simulink model "TestWindRacingDynamicModelRealForce"  (R2022b)
settings: Solver=FixedStepAuto  StartTime=0.0  StopTime=137  FixedStep=simulator.TimeStep  RelTol=1e-3
undefined symbols (not defined in the file): simulator
settings Model: Creator=At  LastModifiedBy=ateay
settings SolverCC: ConcurrentTasks=on  AlgebraicLoopSolver=TrustRegion  InsertRTBMode=Never (minimum delay)
settings DataIOCC: ReturnWorkspaceOutputs=off
settings DebuggingCC: UnconnectedInputMsg=warning  UnconnectedOutputMsg=warning  UnconnectedLineMsg=warning  SFMachineParentedDataDiag=warning  ArithmeticOperatorsInVariantConditions=warning
settings ModelReferenceCC: EnableRefExpFcnMdlSchedulingChecks=on
settings SFSimCC: SimUseLocalCustomCode=off  CustomCodeUndefinedFunction=UseInterfaceOnly
settings RTWCC: RTWUseLocalCustomCode=off
settings CodeAppCC: StateflowObjectComments=on

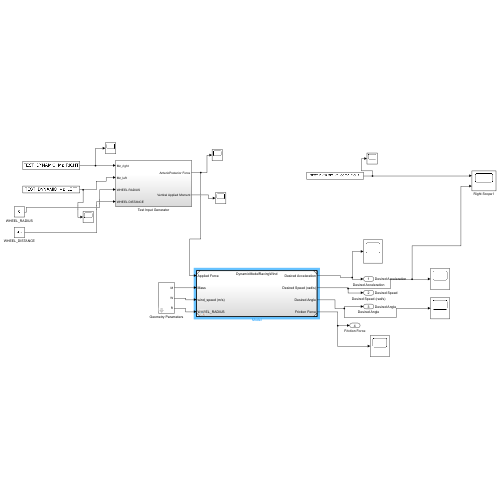
[thumbnail: Simulink's stored preview of the top-level diagram]
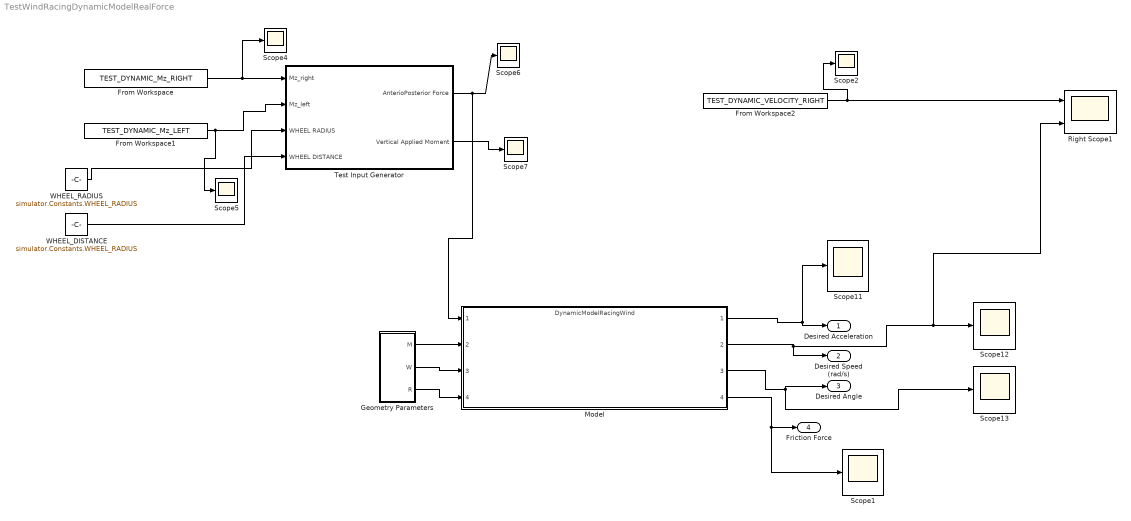
== system TestWindRacingDynamicModelRealForce ==
  From Workspace : FromWorkspace  VariableName=TEST_DYNAMIC_Mz_RIGHT
  From Workspace1 : FromWorkspace  VariableName=TEST_DYNAMIC_Mz_LEFT
  From Workspace2 : FromWorkspace  VariableName=TEST_DYNAMIC_VELOCITY_RIGHT
  Geometry Parameters : Subsystem  mask{M=simulator.Sim.Dynamics.Mass, W=simulator.Sim.Dynamics.wind_speed, rR=simulator.Constants.WHEEL_RADIUS}
      mask prompts: M "Mass"; W "Wind"; rR "Radius"
      mask TypeOptions M: Mass/Value
      mask TypeOptions rR: rR/Value
  Model : ModelReference  ModelNameDialog=DynamicModelRacingWind.slx  SimulationMode=Normal  ModelReferenceVersion=1.17
  Right Scope1 : Scope  NumInputPorts=2
  Scope{1..2,4..7,11..13} (9 alike) : Scope
  Test Input Generator : Subsystem
  WHEEL_DISTANCE : Constant  Value=simulator.Constants.WHEEL_RADIUS
  WHEEL_RADIUS : Constant  Value=simulator.Constants.WHEEL_RADIUS
  Desired Acceleration : Outport  SignalName=Desired Acceleration
  Desired Speed (rad/s) : Outport  Port=2  SignalName=Desired Speed
  Desired Angle : Outport  Port=3  SignalName=Desired Angle
  Friction Force : Outport  Port=4
  wires:
  WHEEL_RADIUS/1 -> Test Input Generator/3(WHEEL RADIUS)
  WHEEL_DISTANCE/1 -> Test Input Generator/4(WHEEL DISTANCE)
  Test Input Generator/1(AnterioPosterior Force) -> Scope6/1, Model/1
  Test Input Generator/2(Vertical Applied Moment) -> Scope7/1
  From Workspace/1 -> Scope4/1, Test Input Generator/1(Mz_right)
  From Workspace1/1 -> Scope5/1, Test Input Generator/2(Mz_left)
  From Workspace2/1 -> Scope2/1, Right Scope1/1
  Geometry Parameters/1(M) -> Model/2
  Geometry Parameters/2(W) -> Model/3
  Geometry Parameters/3(R) -> Model/4
  Model/3 -> Desired Angle/1, Scope13/1
  Model/2 -> Desired Speed (rad/s)/1, Right Scope1/2, Scope12/1
  Model/1 -> Desired Acceleration/1, Scope11/1
  Model/4 -> Scope1/1, Friction Force/1

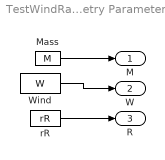
== system TestWindRacingDynamicModelRealForce/Geometry Parameters ==
  Mass : Constant  Value=M
  Wind : Constant  Value=W
  rR : Constant  Value=rR
  M : Outport
  W : Outport  Port=2
  R : Outport  Port=3
  wires:
  Wind/1 -> W/1
  Mass/1 -> M/1
  rR/1 -> R/1

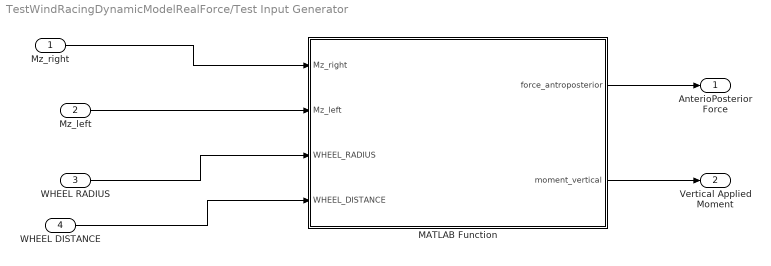
== system TestWindRacingDynamicModelRealForce/Test Input Generator ==
  Mz_right : Inport
  Mz_left : Inport  Port=2
  WHEEL RADIUS : Inport  Port=3
  WHEEL DISTANCE : Inport  Port=4
  MATLAB Function : MATLAB Function  TreatAsAtomicUnit=on
  AnterioPosterior Force : Outport
  Vertical Applied Moment : Outport  Port=2
  wires:
  Mz_right/1 -> MATLAB Function/1(Mz_right)
  Mz_left/1 -> MATLAB Function/2(Mz_left)
  WHEEL RADIUS/1 -> MATLAB Function/3(WHEEL_RADIUS)
  WHEEL DISTANCE/1 -> MATLAB Function/4(WHEEL_DISTANCE)
  MATLAB Function/1(force_antroposterior) -> AnterioPosterior Force/1
  MATLAB Function/2(moment_vertical) -> Vertical Applied Moment/1

== matlab function TestWindRacingDynamicModelRealForce/Test Input Generator/MATLAB Function ==
  data: Mz_right input; Mz_left input; WHEEL_RADIUS input; force_antroposterior output; WHEEL_DISTANCE input; moment_vertical output
function [force_antroposterior,moment_vertical]=Force_Conversion(Mz_right, Mz_left,WHEEL_RADIUS,WHEEL_DISTANCE)

%% This function estimates the force and moment applied at the position of installed force cell,...
...based on the moment applied on the right and left instrumented wheels
    
force_antroposterior=(Mz_right/WHEEL_RADIUS)+(Mz_left/WHEEL_RADIUS);
moment_vertical=((Mz_left/WHEEL_RADIUS)-(Mz_right/WHEEL_RADIUS))*(WHEEL_DISTANCE/2);
